simulink model "z3"  (R2021a)
settings: Solver=VariableStepAuto  StartTime=0.0  StopTime=50.0  RelTol=1e-3
values from neighbouring files (symbols this model uses):
  T = 0.5    [z3_czas_probkowania_T.m]    (also in z9_czas_probkowania_T_wartosc_ud.m = 1)
settings Model: Creator=48604  LastModifiedBy=48604

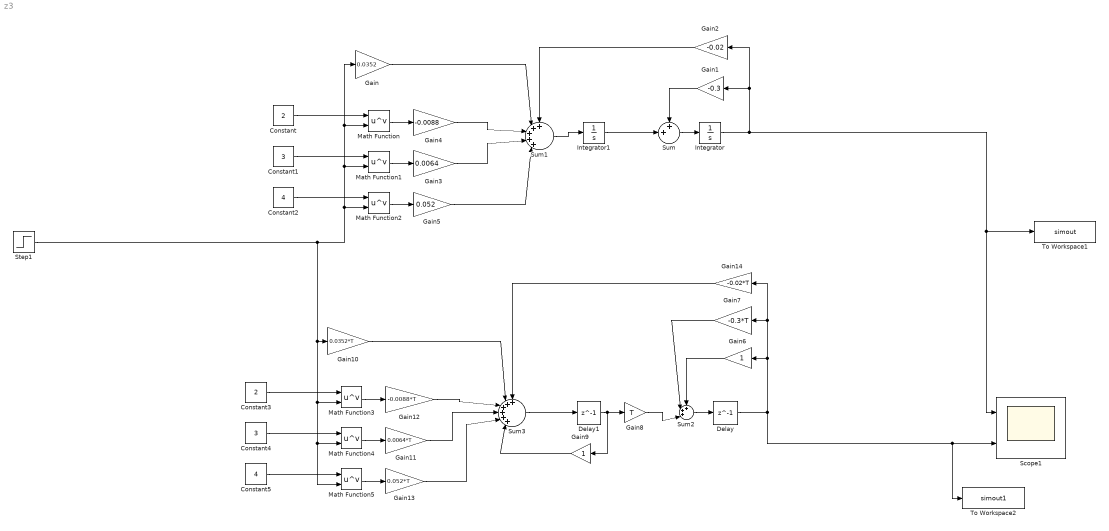
== system z3 ==
  Constant : Constant  Value=2
  Constant1 : Constant  Value=3
  Constant2 : Constant  Value=4
  Constant3 : Constant  Value=2
  Constant4 : Constant  Value=3
  Constant5 : Constant  Value=4
  Delay : Delay  DelayLength=1  InitialCondition=0  SampleTime=0.5
  Delay1 : Delay  DelayLength=1  InitialCondition=0  SampleTime=0.5
  Gain : Gain  Gain=0.0352
  Gain1 : Gain  Gain=-0.3
  Gain10 : Gain  Gain=0.0352*T
  Gain11 : Gain  Gain=0.0064*T
  Gain12 : Gain  Gain=-0.0088*T
  Gain13 : Gain  Gain=0.052*T
  Gain14 : Gain  Gain=-0.02*T
  Gain2 : Gain  Gain=-0.02
  Gain3 : Gain  Gain=0.0064
  Gain4 : Gain  Gain=-0.0088
  Gain5 : Gain  Gain=0.052
  Gain6 : Gain
  Gain7 : Gain  Gain=-0.3*T
  Gain8 : Gain  Gain=T
  Gain9 : Gain
  Integrator : Integrator
  Integrator1 : Integrator
  Math Function{,1..5} (6 alike) : Math  Operator=pow  SaturateOnIntegerOverflow=on
  Scope1 : Scope  NumInputPorts=2
  Step1 : Step  SampleTime=0.5
  Sum : Sum  Inputs=++|
  Sum1 : Sum  Inputs=+++++|
  Sum2 : Sum  Inputs=+++|
  Sum3 : Sum  Inputs=++++++|
  To Workspace1 : ToWorkspace  VariableName=simout  SaveFormat=Structure With Time  SampleTime=-1
  To Workspace2 : ToWorkspace  VariableName=simout1  SaveFormat=Structure With Time  SampleTime=0.1
  wires:
  Integrator1/1 -> Sum/2
  Sum/1 -> Integrator/1
  Integrator/1 -> Scope1/1, To Workspace1/1, Gain2/1, Gain1/1
  Gain1/1 -> Sum/1
  Sum1/1 -> Integrator1/1
  Math Function1/1 -> Gain3/1
  Math Function2/1 -> Gain5/1
  Constant/1 -> Math Function/1
  Constant1/1 -> Math Function1/1
  Constant2/1 -> Math Function2/1
  Step1/1 -> Gain/1, Math Function/2, Math Function1/2, Math Function2/2, Math Function5/2, Math Function4/2, Math Function3/2, Gain10/1
  Gain/1 -> Sum1/2
  Math Function/1 -> Gain4/1
  Gain4/1 -> Sum1/3
  Gain3/1 -> Sum1/4
  Gain5/1 -> Sum1/5
  Gain2/1 -> Sum1/1
  Gain10/1 -> Sum3/2
  Gain9/1 -> Sum3/6
  Gain14/1 -> Sum3/1
  Sum3/1 -> Delay1/1
  Constant4/1 -> Math Function4/1
  Math Function5/1 -> Gain13/1
  Gain12/1 -> Sum3/3
  Math Function4/1 -> Gain11/1
  Constant3/1 -> Math Function3/1
  Constant5/1 -> Math Function5/1
  Sum2/1 -> Delay/1
  Delay/1 -> To Workspace2/1, Scope1/2, Gain7/1, Gain14/1, Gain6/1
  Gain13/1 -> Sum3/5
  Gain6/1 -> Sum2/1
  Gain7/1 -> Sum2/2
  Gain11/1 -> Sum3/4
  Math Function3/1 -> Gain12/1
  Gain8/1 -> Sum2/3
  Delay1/1 -> Gain9/1, Gain8/1
